simulink model "simpleImpControl"  (R2015b)
settings: Solver=VariableStepAuto  StartTime=0.0  StopTime=10.0  RelTol=1e-3
values from neighbouring files (symbols this model uses):
  dt = 0.01    [learnPolicyFcn.m]
  Kd = 2*zeta.*sqrt((Kp + Kp_env))    [computeDamping.m]
  Kp = diag([Kp(1), Kp(2), Kp(2), 300, 300, 300])    [computeDamping.m]
  Kp_env = diag(Kp_env)    [computeDamping.m]    (also in learnPolicyFcn.m = [1e4, 1e4, 1e4, 0, 0, 0])
  q0 = robot.ikine(T0,q0_est,[1 1 0 0 0 1])    [genInitTrajectory.m]    (also in genTrajectory.m = robot.ikine(T0,q0_est,[1 1 0 0 0 1],'pinv'))
  robot = SerialLink([link1, link2, link3], 'name', '3link-robot',     'base',[eye(3), zeros(3,1); zeros(1,3), 1], 'qlim',[-pi, pi; -pi, pi; -pi, pi],     'tool',[eye(3), zeros(3,1); zeros(1,3), 1])    [init_3Lbot.m]    (also in init_puma.m = p560)
  xc = [0.65, 10, 10, 10, 10, 10]'    [learnPolicyFcn.m]
undefined symbols (not defined in the file or in its folder): maniplty
libraries: roblocks x9
settings Model: Creator=victor  LastModifiedBy=victor

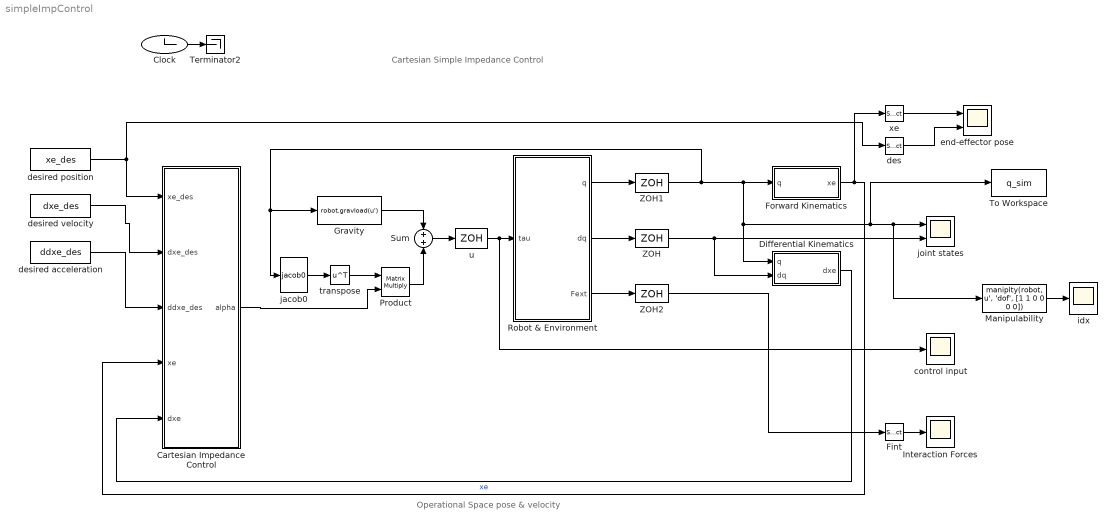
== system simpleImpControl ==
  note: Operational Space pose & velocity
  note: Cartesian Simple Impedance Control
  Cartesian Impedance Control : Subsystem
  Clock : Clock
  Differential Kinematics : Subsystem
  Fint : Selector  InputPortWidth=6  IndexOptions=Index vector (dialog)  Indices=[1 2]  OutputSizes=1
  Forward Kinematics : Subsystem
  Gravity : MATLABFcn  MATLABFcn=robot.gravload(u')  Output1D=off
  Interaction Forces : Scope
  Manipulability : MATLABFcn  MATLABFcn=maniplty(robot, u', 'dof', [1 1 0 0 0 0])
  Product : Product  Multiplication=Matrix(*)
  Robot & Environment : Subsystem
  Sum : Sum
  Terminator2 : Terminator
  To Workspace : ToWorkspace  VariableName=q_sim  SaveFormat=Timeseries  SampleTime=dt
  ZOH : ZeroOrderHold  SampleTime=dt
  ZOH1 : ZeroOrderHold  SampleTime=dt
  ZOH2 : ZeroOrderHold  SampleTime=dt
  control input : Scope
  des : Selector  InputPortWidth=6  IndexOptions=Index vector (dialog)  Indices=[1 2 6]  OutputSizes=1
  desired acceleration : FromWorkspace  VariableName=ddxe_des  SampleTime=dt
  desired position : FromWorkspace  VariableName=xe_des  SampleTime=dt
  desired velocity : FromWorkspace  VariableName=dxe_des  SampleTime=dt
  end-effector pose : Scope  NumInputPorts=2
  idx : Scope
  "jacob0 " : roblocks/Kinematics/jacob0   robot=robot
  joint states : Scope  NumInputPorts=2
  transpose : Math  Operator=transpose  SaturateOnIntegerOverflow=on
  u : ZeroOrderHold  SampleTime=dt
  xe : Selector  InputPortWidth=6  IndexOptions=Index vector (dialog)  Indices=[1 2 6]  OutputSizes=1
  wires:
  Sum/1 -> u/1
  u/1 -> control input/1, Robot & Environment/1(tau)
  Clock/1 -> Terminator2/1
  desired position/1 -> des/1, Cartesian Impedance Control/1(xe_des)
  desired velocity/1 -> Cartesian Impedance Control/2(dxe_des)
  desired acceleration/1 -> Cartesian Impedance Control/3(ddxe_des)
  Robot & Environment/1(q) -> ZOH1/1
  Robot & Environment/2(dq) -> ZOH/1
  Robot & Environment/3(Fext) -> ZOH2/1
  Differential Kinematics/1(dxe) -> Cartesian Impedance Control/5(dxe)
  Forward Kinematics/1(xe) -> xe/1, Cartesian Impedance Control/4(xe)  "xe"
  ZOH2/1 -> Fint/1
  xe/1 -> end-effector pose/1
  des/1 -> end-effector pose/2
  Fint/1 -> Interaction Forces/1
  ZOH/1 -> joint states/2, Differential Kinematics/2(dq)
  ZOH1/1 -> "jacob0 "/1, Gravity/1, Differential Kinematics/1(q), Manipulability/1, joint states/1, To Workspace/1, Forward Kinematics/1(q)
  Manipulability/1 -> idx/1
  "jacob0 "/1 -> transpose/1
  transpose/1 -> Product/1
  Gravity/1 -> Sum/1
  Cartesian Impedance Control/1(alpha) -> Product/2
  Product/1 -> Sum/2

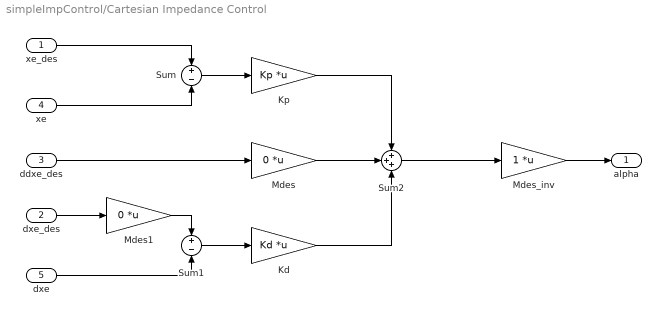
== system simpleImpControl/Cartesian Impedance Control ==
  xe_des : Inport
  dxe_des : Inport  Port=2
  ddxe_des : Inport  Port=3
  xe : Inport  Port=4
  dxe : Inport  Port=5
  Kd : Gain  Gain=Kd  Multiplication=Matrix(K*u)  SaturateOnIntegerOverflow=on  OutDataTypeStr=Inherit: Same as input  ParamDataTypeStr=Inherit: Same as input
  Kp : Gain  Gain=Kp  Multiplication=Matrix(K*u)  SaturateOnIntegerOverflow=on  OutDataTypeStr=Inherit: Same as input  ParamDataTypeStr=Inherit: Same as input
  Mdes : Gain  Gain=0  Multiplication=Matrix(K*u)  SaturateOnIntegerOverflow=on  OutDataTypeStr=Inherit: Same as input  ParamDataTypeStr=Inherit: Same as input
  Mdes1 : Gain  Gain=0  Multiplication=Matrix(K*u)  SaturateOnIntegerOverflow=on  OutDataTypeStr=Inherit: Same as input  ParamDataTypeStr=Inherit: Same as input
  Mdes_inv : Gain  Multiplication=Matrix(K*u)  SaturateOnIntegerOverflow=on  OutDataTypeStr=Inherit: Same as input  ParamDataTypeStr=Inherit: Same as input
  Sum : Sum  Inputs=+-  SaturateOnIntegerOverflow=on  InputSameDT=on  OutDataTypeStr=Inherit: Same as first input
  Sum1 : Sum  Inputs=+-  SaturateOnIntegerOverflow=on  InputSameDT=on  OutDataTypeStr=Inherit: Same as first input
  Sum2 : Sum  Inputs=+++  SaturateOnIntegerOverflow=on  InputSameDT=on  OutDataTypeStr=Inherit: Same as first input
  alpha : Outport
  wires:
  Sum/1 -> Kp/1
  Kp/1 -> Sum2/1
  Kd/1 -> Sum2/3
  Sum2/1 -> Mdes_inv/1
  xe_des/1 -> Sum/1
  Sum1/1 -> Kd/1
  Mdes/1 -> Sum2/2
  Mdes_inv/1 -> alpha/1
  dxe/1 -> Sum1/2
  xe/1 -> Sum/2
  dxe_des/1 -> Mdes1/1
  ddxe_des/1 -> Mdes/1
  Mdes1/1 -> Sum1/1

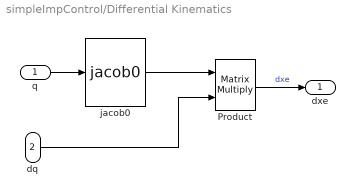
== system simpleImpControl/Differential Kinematics ==
  q : Inport
  dq : Inport  Port=2
  Product : Product  Multiplication=Matrix(*)
  "jacob0 " : roblocks/Kinematics/jacob0   robot=robot
  dxe : Outport
  wires:
  "jacob0 "/1 -> Product/1
  q/1 -> "jacob0 "/1
  Product/1 -> dxe/1  "dxe"
  dq/1 -> Product/2

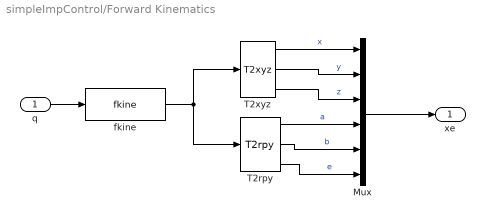
== system simpleImpControl/Forward Kinematics ==
  q : Inport
  Mux : Mux  Inputs=6
  T2rpy : roblocks/Transform Conversion/T2rpy
  T2xyz : roblocks/Transform Conversion/T2xyz
  fkine : roblocks/Kinematics/fkine  robot=robot
  xe : Outport
  wires:
  T2xyz/3 -> Mux/3  "z"
  T2rpy/3 -> Mux/6  "e"
  T2rpy/1 -> Mux/4  "a"
  T2xyz/2 -> Mux/2  "y"
  q/1 -> fkine/1
  fkine/1 -> T2rpy/1, T2xyz/1
  T2xyz/1 -> Mux/1  "x"
  T2rpy/2 -> Mux/5  "b"
  Mux/1 -> xe/1

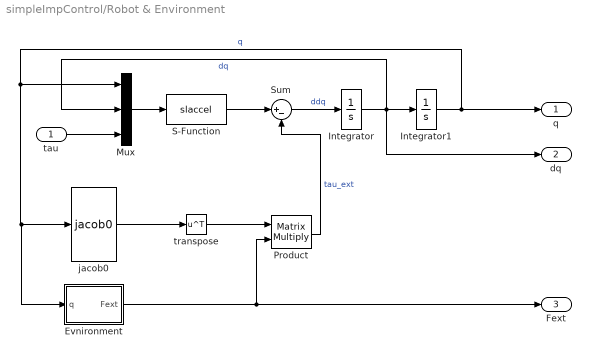
== system simpleImpControl/Robot & Environment ==
  tau : Inport
  Evnironment : Subsystem
  Integrator : Integrator
  Integrator1 : Integrator  InitialCondition=q0
  Mux : Mux  Inputs=3
  Product : Product  Multiplication=Matrix(*)
  S-Function : S-Function  FunctionName=slaccel  Parameters=robot  SFunctionDeploymentMode=off  EnableBusSupport=off
  Sum : Sum  Inputs=|+-
  "jacob0 " : roblocks/Kinematics/jacob0   robot=robot
      link override MATLAB Fcn: MATLABFcn=jacob0(robot,u, 'rpy')
  transpose : Math  Operator=transpose  SaturateOnIntegerOverflow=on
  q : Outport
  dq : Outport  Port=2
  Fext : Outport  Port=3
  wires:
  S-Function/1 -> Sum/1
  Mux/1 -> S-Function/1
  Integrator/1 -> Mux/2, Integrator1/1, dq/1  "dq"
  tau/1 -> Mux/3
  "jacob0 "/1 -> transpose/1
  Product/1 -> Sum/2  "tau_ext"
  Evnironment/1(Fext) -> Fext/1, Product/2
  Integrator1/1 -> "jacob0 "/1, Evnironment/1(q), Mux/1, q/1  "q"
  Sum/1 -> Integrator/1  "ddq"
  transpose/1 -> Product/1

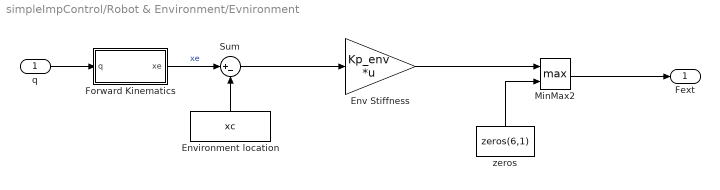
== system simpleImpControl/Robot & Environment/Evnironment ==
  q : Inport
  Env Stiffness : Gain  Gain=Kp_env  Multiplication=Matrix(K*u)
  Environment location : Constant  Value=xc  SampleTime=dt
  Forward Kinematics : Subsystem
  MinMax2 : MinMax  Function=max  Inputs=2
  Sum : Sum  Inputs=|+-
  zeros : Constant  Value=zeros(6,1)  SampleTime=dt
  Fext : Outport
  wires:
  Environment location/1 -> Sum/2
  q/1 -> Forward Kinematics/1(q)
  Sum/1 -> Env Stiffness/1
  Env Stiffness/1 -> MinMax2/1
  zeros/1 -> MinMax2/2
  MinMax2/1 -> Fext/1
  Forward Kinematics/1(xe) -> Sum/1  "xe"

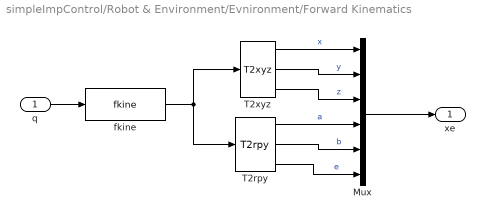
== system simpleImpControl/Robot & Environment/Evnironment/Forward Kinematics ==
  q : Inport
  Mux : Mux  Inputs=6
  T2rpy : roblocks/Transform Conversion/T2rpy
  T2xyz : roblocks/Transform Conversion/T2xyz
  fkine : roblocks/Kinematics/fkine  robot=robot
  xe : Outport
  wires:
  T2xyz/3 -> Mux/3  "z"
  T2rpy/3 -> Mux/6  "e"
  T2rpy/1 -> Mux/4  "a"
  T2xyz/2 -> Mux/2  "y"
  q/1 -> fkine/1
  fkine/1 -> T2rpy/1, T2xyz/1
  T2xyz/1 -> Mux/1  "x"
  T2rpy/2 -> Mux/5  "b"
  Mux/1 -> xe/1
